simulink model "Turtle_RRT_Algorithm"  (R2023a)
settings: Solver=FixedStepDiscrete  StartTime=0.0  StopTime=Inf  FixedStep=0.01  RelTol=1e-3  EnableMultiTasking=on
model workspace (MAT data in the model file):
  SL_ROS_VariableLengthArrays_MaxSizes.CommonInfo.ArrayTruncateAction = 'EmitWarning'
  SL_ROS_VariableLengthArrays_MaxSizes.MsgTypeMap = containers.Map
  SL_ROS_VariableLengthArrays_MaxSizes.MsgTypeMap.serialization.keys = {'sensor_msgs/LaserScan'}
  SL_ROS_VariableLengthArrays_MaxSizes.MsgTypeMap.serialization.values{1}(1).PropertyName = 'Intensities'
  SL_ROS_VariableLengthArrays_MaxSizes.MsgTypeMap.serialization.values{1}(1).DataType = 'single'
  SL_ROS_VariableLengthArrays_MaxSizes.MsgTypeMap.serialization.values{1}(1).MaxLength = 360
  SL_ROS_VariableLengthArrays_MaxSizes.MsgTypeMap.serialization.values{1}(2).PropertyName = 'Ranges'
  SL_ROS_VariableLengthArrays_MaxSizes.MsgTypeMap.serialization.values{1}(2).DataType = 'single'
  SL_ROS_VariableLengthArrays_MaxSizes.MsgTypeMap.serialization.values{1}(2).MaxLength = 360
  SL_ROS_VariableLengthArrays_MaxSizes.MsgTypeMap.serialization.uniformity = 0
  SL_ROS_VariableLengthArrays_MaxSizes.MsgTypeMap.serialization.keyType = 'char'
  SL_ROS_VariableLengthArrays_MaxSizes.MsgTypeMap.serialization.valueType = 'any'
undefined symbols (not defined in the file or in its folder): Angular, gray, Linear
libraries: visiontextngfix x10, robotlib x6, simulink x4
settings Model: Creator=The MathWorks, Inc.  LastModifiedBy=cesf9
settings SolverCC: AlgebraicLoopSolver=TrustRegion
settings DataIOCC: LimitDataPoints=on  SaveFormat=Array  ReturnWorkspaceOutputs=off
settings OptimizationCC: LifeSpan=Inf  MaxStackSize=64
settings DebuggingCC: SolverPrmCheckMsg=warning  MultiTaskRateTransMsg=warning  UnconnectedInputMsg=warning  UnconnectedOutputMsg=warning  UnconnectedLineMsg=warning  SFUnexpectedBacktrackingDiag=warning  SFNoUnconditionalDefaultTransitionDiag=warning  SFExecutionAtInitializationDiag=none  ArithmeticOperatorsInVariantConditions=warning
settings HardwareCC: ProdBitPerPointer=32  ProdBitPerSizeT=32  ProdBitPerPtrDiffT=32  ProdLargestAtomicFloat=None  ProdIntDivRoundTo=Undefined  ProdEndianess=Unspecified  ProdWordSize=32  ProdHWDeviceType=Generic->Unspecified (assume 32-bit Generic)  UseEmbeddedCoderFeatures=off
settings ModelReferenceCC: EnableRefExpFcnMdlSchedulingChecks=on  PropagateSignalLabelsOutOfModel=off
settings SFSimCC: SimUseLocalCustomCode=off  SimTargetLang=C++
settings RTWCC: Description=Embedded Coder  SystemTargetFile=ert.tlc  HardwareBoard=Robot Operating System (ROS)  TLCOptions=-aInlineSetEventsForThisBaseRateFcn=TLC_FALSE -aSuppressMultiTaskScheduler=TLC_FALSE -aRateBasedStepFcn=0  TemplateMakefile=ert_default_tmf  RTWUseLocalCustomCode=off  Toolchain=Catkin  TargetLang=C++
settings CodeAppCC: StateflowObjectComments=on
settings ERTTargetCC: MultiwordLength=2048  ERTCustomFileBanners=off  SupportContinuousTime=on  SupportNonInlinedSFcns=on  RemoveResetFunc=off  SupportVariableSizeSignals=on  ModelStepFunctionPrototypeControlCompliant=off  ConvertIfToSwitch=off  SuppressUnreachableDefaultCases=off
settings ConfigComp: CovMetricSettings=dw  CovSaveCumulativeToWorkspaceVar=on  CovSaveSingleToWorkspaceVar=on  CovExternalEMLEnable=off  CovSFcnEnable=off

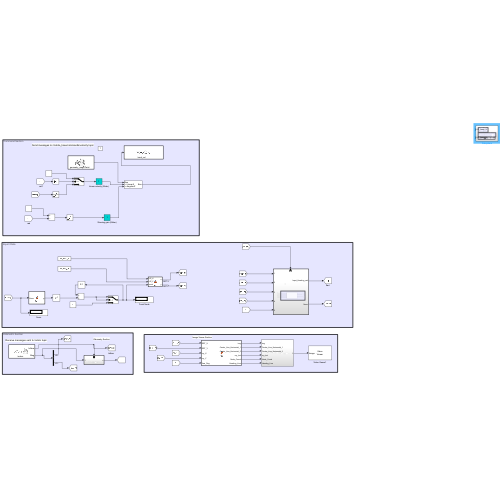
[thumbnail: Simulink's stored preview of the top-level diagram]
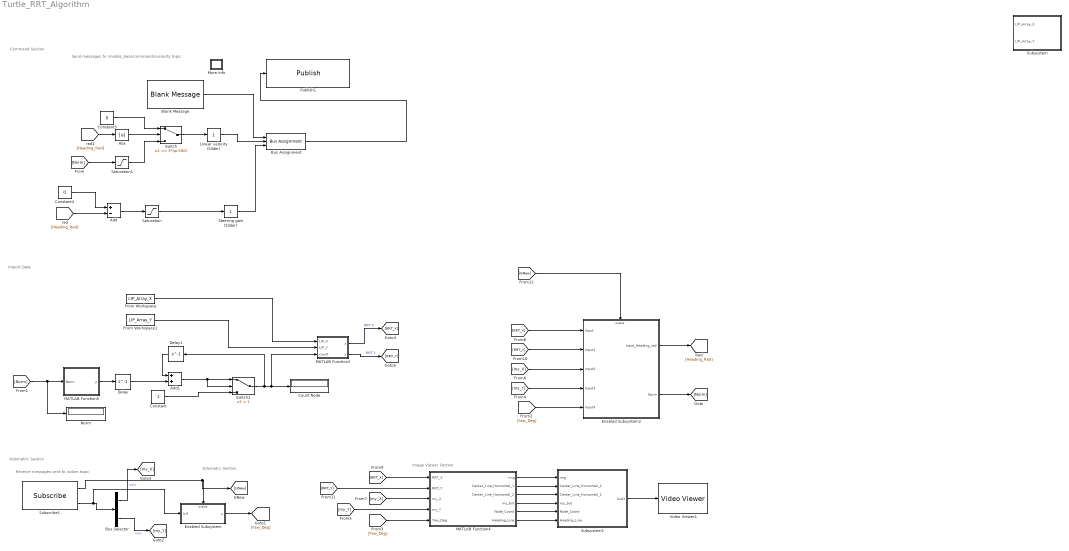
== system Turtle_RRT_Algorithm ==
  note: Image Viewer Section
  note: Import Data
  note: Odometry Section
  note: Odometric Section
  note: Command Section
  note: Receive messages sent to /odom topic
  note: Send messages to /mobile_base/commands/velocity topic
  Abs : Abs  SaturateOnIntegerOverflow=off
  Add : Sum  Inputs=+-
  Add1 : Sum
  Blank Message : robotlib/Blank Message  messageClass=Message  entityType=geometry_msgs/Twist  messageType=geometry_msgs/Twist  SampleTime=0.01  legacyBusStruct=off
  Bus Assignment : BusAssignment  DialogController=Simulink.DDGSource_BusAssignment  AssignedSignals=Linear.X,Angular.Z
  Bus Selector : BusSelector  DialogController=Simulink.DDGSource_BusSelector  OutputSignals=Pose.Pose.Position.X,Pose.Pose.Position.Y
  Constant : Constant
  Constant3 : Constant  Value=0
  Constant4 : Constant  Value=0
  Count Node : Display
  Delay : Delay  DelayLength=1
  Delay1 : Delay  DelayLength=1
  Enabled Subsystem : Subsystem  TreatAsAtomicUnit=on
  Enabled Subsystem2 : Subsystem  TreatAsAtomicUnit=on
  From Workspace : FromWorkspace  VariableName=LIP_Array_X  SampleTime=1
  From Workspace1 : FromWorkspace  VariableName=LIP_Array_Y  SampleTime=1
  Linear velocity (Slider) : simulink/Math Operations/Slider Gain  gain=1  low=0  high=2
  MATLAB Function2 : MATLAB Function  TreatAsAtomicUnit=on
  MATLAB Function4 : MATLAB Function  TreatAsAtomicUnit=on
  MATLAB Function5 : MATLAB Function  TreatAsAtomicUnit=on
  More Info : Subsystem
      settings: OpenFcn=showdemo(bdroot(gcb))
      mask Display: disp('?')
  Norm : Display
  Publish1 : robotlib/Publish  topicSource=Select from ROS network  topic=/cmd_vel  messageType=geometry_msgs/Twist  legacyBusStruct=off  messageQueueLength=105
  Saturation : Saturate  UpperLimit=0.3  LowerLimit=-0.3
  Saturation1 : Saturate  UpperLimit=0.3  LowerLimit=-0.3
  Steering gain (Slider) : simulink/Math Operations/Slider Gain  gain=1  low=-1  high=1
  Subscribe1 : robotlib/Subscribe  topicSource=Select from ROS network  topic=/odom  messageType=nav_msgs/Odometry  SampleTime=-1  legacyBusStruct=off  messageQueueLength=51
  Subsystem : Subsystem
  Subsystem1 : Subsystem
  Switch : Switch  Threshold=5*(pi/180)  SaturateOnIntegerOverflow=off  InputSameDT=off
  Switch1 : Switch  Criteria=u2 > Threshold  Threshold=1  SaturateOnIntegerOverflow=off  InputSameDT=off
  Video Viewer1 : VideoViewer  colormapValue=gray(256)  FigPos=[138 1038 776 784]
  wires:
  Subscribe1/2 -> Enabled Subsystem/1(In3), Bus Selector/1
  Subscribe1/1 -> [IsNew], Enabled Subsystem/Enable
  Steering gain (Slider)/1 -> Bus Assignment/3
  Bus Assignment/1 -> Publish1/1
  Blank Message/1 -> Bus Assignment/1
  Linear velocity (Slider)/1 -> Bus Assignment/2
  From Workspace/1 -> MATLAB Function2/1(LIP_X)
  From Workspace1/1 -> MATLAB Function2/2(LIP_Y)
  Switch/1 -> Linear velocity (Slider)/1
  MATLAB Function4/1(img) -> Subsystem1/1(img)
  MATLAB Function4/2(Center_Line_Horizontal_1) -> Subsystem1/2(Center_Line_Horizontal_1)
  MATLAB Function4/3(Center_Line_Horizontal_2) -> Subsystem1/3(Center_Line_Horizontal_2)
  MATLAB Function4/4(my_bot) -> Subsystem1/4(my_bot)
  MATLAB Function4/5(Node_Coord) -> Subsystem1/5(Node_Coord)
  Subsystem1/1(Out1) -> Video Viewer1/1
  MATLAB Function4/6(Heading_Line) -> Subsystem1/6(Heading_Line)
  Saturation/1 -> Steering gain (Slider)/1
  Constant4/1 -> Add/1
  Add/1 -> Saturation/1
  MATLAB Function5/1(p) -> Delay/1
  Delay/1 -> Add1/2
  Add1/1 -> Switch1/1, Switch1/2
  Constant/1 -> Switch1/3
  Switch1/1 -> MATLAB Function2/3(count), Count Node/1, Delay1/1
  Delay1/1 -> Add1/1
  Abs/1 -> Switch/2
  [Heading_Rad] -> Add/2
  [Norm] -> Saturation1/1
  [Norm] -> Norm/1, MATLAB Function5/1(Norm)
  Enabled Subsystem/1(u) -> [Yaw_Deg]
  [Yaw_Deg] -> MATLAB Function4/5(Yaw_Deg)
  Bus Selector/2 -> [my_Y]  "<Y>"
  [my_Y] -> MATLAB Function4/4(my_Y)
  Bus Selector/1 -> [my_X]  "<X>"
  [my_X] -> MATLAB Function4/3(my_X)
  MATLAB Function2/1(x) -> [RRT_X]  "RRT X"
  [RRT_X] -> MATLAB Function4/1(RRT_X)
  MATLAB Function2/2(y) -> [RRT_Y]  "RRT Y"
  [RRT_Y] -> MATLAB Function4/2(RRT_Y)
  Enabled Subsystem2/1(Input_Heading_rad) -> [Heading_Rad]
  Enabled Subsystem2/2(Norm) -> [Norm]
  [RRT_X] -> Enabled Subsystem2/1(Input)
  [RRT_Y] -> Enabled Subsystem2/2(Input1)
  [my_X] -> Enabled Subsystem2/3(Input2)
  [my_Y] -> Enabled Subsystem2/4(Input3)
  [Yaw_Deg] -> Enabled Subsystem2/5(Input4)
  [IsNew] -> Enabled Subsystem2/Enable
  [Heading_Rad] -> Abs/1
  Saturation1/1 -> Switch/3
  Constant3/1 -> Switch/1

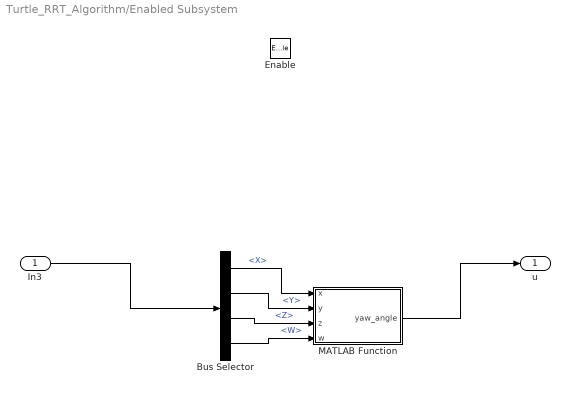
== system Turtle_RRT_Algorithm/Enabled Subsystem ==
  In3 : Inport
  Enable : EnablePort
  Bus Selector : BusSelector  OutputSignals=Pose.Pose.Orientation.X,Pose.Pose.Orientation.Y,Pose.Pose.Orientation.Z,Pose.Pose.Orientation.W
  MATLAB Function : MATLAB Function  TreatAsAtomicUnit=on
  u : Outport
  wires:
  In3/1 -> Bus Selector/1
  Bus Selector/1 -> MATLAB Function/1(x)  "<X>"
  Bus Selector/2 -> MATLAB Function/2(y)  "<Y>"
  Bus Selector/3 -> MATLAB Function/3(z)  "<Z>"
  Bus Selector/4 -> MATLAB Function/4(w)  "<W>"
  MATLAB Function/1(yaw_angle) -> u/1

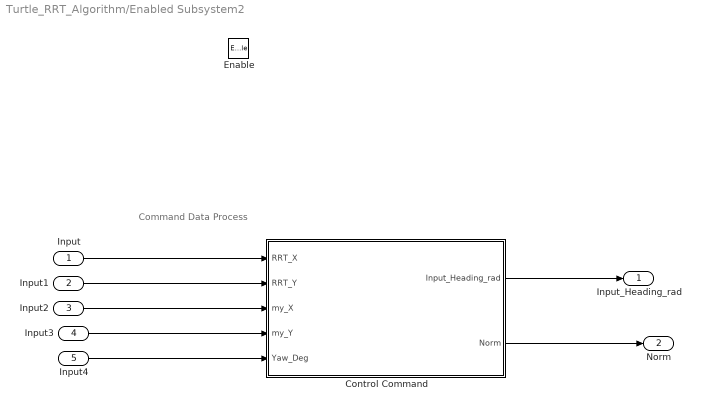
== system Turtle_RRT_Algorithm/Enabled Subsystem2 ==
  note: Command Data Process
  Input : Inport
  Input1 : Inport  Port=2
  Input2 : Inport  Port=3
  Input3 : Inport  Port=4
  Input4 : Inport  Port=5
  Enable : EnablePort
  Control Command : MATLAB Function  TreatAsAtomicUnit=on
  Input_Heading_rad : Outport
  Norm : Outport  Port=2
  wires:
  Control Command/1(Input_Heading_rad) -> Input_Heading_rad/1
  Input4/1 -> Control Command/5(Yaw_Deg)
  Input2/1 -> Control Command/3(my_X)
  Control Command/2(Norm) -> Norm/1
  Input/1 -> Control Command/1(RRT_X)
  Input3/1 -> Control Command/4(my_Y)
  Input1/1 -> Control Command/2(RRT_Y)

== system Turtle_RRT_Algorithm/More Info ==

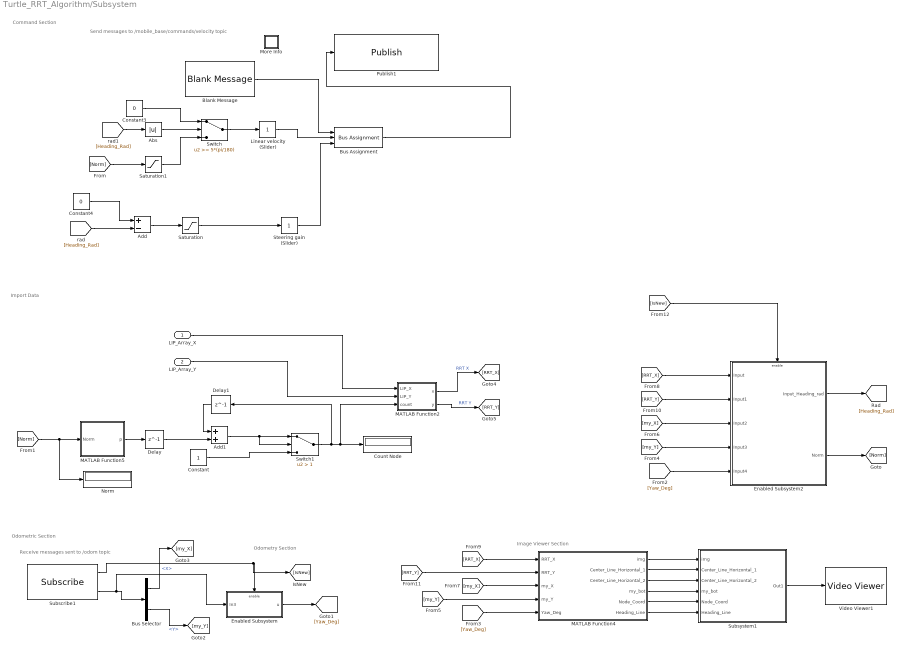
== system Turtle_RRT_Algorithm/Subsystem ==
  note: Command Section
  note: Odometry Section
  note: Image Viewer Section
  note: Import Data
  note: Odometric Section
  note: Receive messages sent to /odom topic
  note: Send messages to /mobile_base/commands/velocity topic
  LIP_Array_X : Inport
  LIP_Array_Y : Inport  Port=2
  Abs : Abs  SaturateOnIntegerOverflow=off
  Add : Sum  Inputs=+-
  Add1 : Sum
  Blank Message : robotlib/Blank Message  messageClass=Message  entityType=geometry_msgs/Twist  messageType=geometry_msgs/Twist  SampleTime=0.01  legacyBusStruct=off
  Bus Assignment : BusAssignment  DialogController=Simulink.DDGSource_BusAssignment  AssignedSignals=Linear.X,Angular.Z
  Bus Selector : BusSelector  DialogController=Simulink.DDGSource_BusSelector  OutputSignals=Pose.Pose.Position.X,Pose.Pose.Position.Y
  Constant : Constant
  Constant3 : Constant  Value=0
  Constant4 : Constant  Value=0
  Count Node : Display
  Delay : Delay  DelayLength=1
  Delay1 : Delay  DelayLength=1
  Enabled Subsystem : Subsystem  TreatAsAtomicUnit=on
  Enabled Subsystem2 : Subsystem  TreatAsAtomicUnit=on
  Linear velocity (Slider) : simulink/Math Operations/Slider Gain  gain=1  low=0  high=2
  MATLAB Function2 : MATLAB Function  TreatAsAtomicUnit=on
  MATLAB Function4 : MATLAB Function  TreatAsAtomicUnit=on
  MATLAB Function5 : MATLAB Function  TreatAsAtomicUnit=on
  More Info : Subsystem
      settings: OpenFcn=showdemo(bdroot(gcb))
      mask Display: disp('?')
  Norm : Display
  Publish1 : robotlib/Publish  topicSource=Select from ROS network  topic=/cmd_vel  messageType=geometry_msgs/Twist  legacyBusStruct=off  messageQueueLength=105
  Saturation : Saturate  UpperLimit=0.3  LowerLimit=-0.3
  Saturation1 : Saturate  UpperLimit=0.3  LowerLimit=-0.3
  Steering gain (Slider) : simulink/Math Operations/Slider Gain  gain=1  low=-1  high=1
  Subscribe1 : robotlib/Subscribe  topicSource=Select from ROS network  topic=/odom  messageType=nav_msgs/Odometry  SampleTime=-1  legacyBusStruct=off  messageQueueLength=51
  Subsystem1 : Subsystem
  Switch : Switch  Threshold=5*(pi/180)  SaturateOnIntegerOverflow=off  InputSameDT=off
  Switch1 : Switch  Criteria=u2 > Threshold  Threshold=1  SaturateOnIntegerOverflow=off  InputSameDT=off
  Video Viewer1 : VideoViewer  colormapValue=gray(256)  FigPos=[138 1038 776 784]
  wires:
  Saturation/1 -> Steering gain (Slider)/1
  Subsystem1/1(Out1) -> Video Viewer1/1
  [Norm] -> Saturation1/1
  [Heading_Rad] -> Add/2
  Enabled Subsystem/1(u) -> [Yaw_Deg]
  Delay1/1 -> Add1/1
  MATLAB Function4/1(img) -> Subsystem1/1(img)
  Bus Selector/2 -> [my_Y]  "<Y>"
  [Yaw_Deg] -> MATLAB Function4/5(Yaw_Deg)
  Add/1 -> Saturation/1
  Subscribe1/2 -> Enabled Subsystem/1(In3), Bus Selector/1
  Steering gain (Slider)/1 -> Bus Assignment/3
  Switch/1 -> Linear velocity (Slider)/1
  Bus Assignment/1 -> Publish1/1
  MATLAB Function4/5(Node_Coord) -> Subsystem1/5(Node_Coord)
  [my_X] -> Enabled Subsystem2/3(Input2)
  Blank Message/1 -> Bus Assignment/1
  MATLAB Function4/4(my_bot) -> Subsystem1/4(my_bot)
  LIP_Array_X/1 -> MATLAB Function2/1(LIP_X)
  MATLAB Function4/3(Center_Line_Horizontal_2) -> Subsystem1/3(Center_Line_Horizontal_2)
  Bus Selector/1 -> [my_X]  "<X>"
  MATLAB Function5/1(p) -> Delay/1
  Add1/1 -> Switch1/1, Switch1/2
  [my_X] -> MATLAB Function4/3(my_X)
  [RRT_X] -> MATLAB Function4/1(RRT_X)
  Enabled Subsystem2/2(Norm) -> [Norm]
  [my_Y] -> MATLAB Function4/4(my_Y)
  [Norm] -> Norm/1, MATLAB Function5/1(Norm)
  MATLAB Function2/2(y) -> [RRT_Y]  "RRT Y"
  Enabled Subsystem2/1(Input_Heading_rad) -> [Heading_Rad]
  Delay/1 -> Add1/2
  [IsNew] -> Enabled Subsystem2/Enable
  Subscribe1/1 -> [IsNew], Enabled Subsystem/Enable
  Saturation1/1 -> Switch/3
  Constant/1 -> Switch1/3
  MATLAB Function4/6(Heading_Line) -> Subsystem1/6(Heading_Line)
  [Yaw_Deg] -> Enabled Subsystem2/5(Input4)
  LIP_Array_Y/1 -> MATLAB Function2/2(LIP_Y)
  MATLAB Function2/1(x) -> [RRT_X]  "RRT X"
  Switch1/1 -> MATLAB Function2/3(count), Count Node/1, Delay1/1
  Linear velocity (Slider)/1 -> Bus Assignment/2
  [RRT_X] -> Enabled Subsystem2/1(Input)
  [Heading_Rad] -> Abs/1
  Constant4/1 -> Add/1
  Abs/1 -> Switch/2
  [my_Y] -> Enabled Subsystem2/4(Input3)
  Constant3/1 -> Switch/1
  [RRT_Y] -> Enabled Subsystem2/2(Input1)
  MATLAB Function4/2(Center_Line_Horizontal_1) -> Subsystem1/2(Center_Line_Horizontal_1)
  [RRT_Y] -> MATLAB Function4/2(RRT_Y)

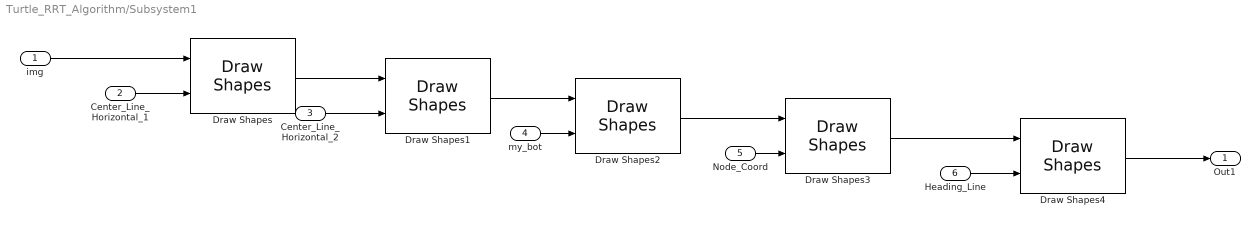
== system Turtle_RRT_Algorithm/Subsystem1 ==
  img : Inport
  Center_Line_Horizontal_1 : Inport  Port=2
  Center_Line_Horizontal_2 : Inport  Port=3
  my_bot : Inport  Port=4
  Node_Coord : Inport  Port=5
  Heading_Line : Inport  Port=6
  Draw Shapes : visiontextngfix/Draw Shapes  shape=Lines  fill=off  lineWidth=1  fillClrSource=Specify via dialog  display=Black  intensity=200  color=[255 0 0]  opacity=0.6  viewport=Entire image  antialiasing=off  inType=Obsolete  imagePorts=One multidimensional signal  roundingMode=Floor  overflowMode=off  memoryMode=Specify word length  memoryWordLength=16  prodOutputMode=Binary point scaling  prodOutputWordLength=32  prodOutputFracLength=14  memoryFracLength=15
  Draw Shapes1 : visiontextngfix/Draw Shapes  shape=Lines  fill=off  lineWidth=1  fillClrSource=Specify via dialog  display=Black  intensity=200  color=[200 255 100]  opacity=0.6  viewport=Entire image  antialiasing=off  inType=Obsolete  imagePorts=One multidimensional signal  roundingMode=Floor  overflowMode=off  memoryMode=Specify word length  memoryWordLength=16  prodOutputMode=Binary point scaling  prodOutputWordLength=32  prodOutputFracLength=14  memoryFracLength=15
  Draw Shapes2 : visiontextngfix/Draw Shapes  shape=Circles  fill=off  lineWidth=3  fillClrSource=Specify via dialog  display=Black  intensity=200  color=[200 255 100]  opacity=0.6  viewport=Entire image  antialiasing=off  inType=Obsolete  imagePorts=One multidimensional signal  roundingMode=Floor  overflowMode=off  memoryMode=Specify word length  memoryWordLength=16  prodOutputMode=Binary point scaling  prodOutputWordLength=32  prodOutputFracLength=14  memoryFracLength=15
  Draw Shapes3 : visiontextngfix/Draw Shapes  shape=Circles  fill=on  lineWidth=1  fillClrSource=Specify via dialog  display=Black  intensity=200  color=[200 255 100]  opacity=0.6  viewport=Entire image  antialiasing=off  inType=Obsolete  imagePorts=One multidimensional signal  roundingMode=Floor  overflowMode=off  memoryMode=Specify word length  memoryWordLength=16  prodOutputMode=Binary point scaling  prodOutputWordLength=32  prodOutputFracLength=14  memoryFracLength=15
  Draw Shapes4 : visiontextngfix/Draw Shapes  shape=Lines  fill=off  lineWidth=1  fillClrSource=Specify via dialog  display=Black  intensity=200  color=[200 255 100]  opacity=0.6  viewport=Entire image  antialiasing=off  inType=Obsolete  imagePorts=One multidimensional signal  roundingMode=Floor  overflowMode=off  memoryMode=Specify word length  memoryWordLength=16  prodOutputMode=Binary point scaling  prodOutputWordLength=32  prodOutputFracLength=14  memoryFracLength=15
  Out1 : Outport
  wires:
  Draw Shapes1/1 -> Draw Shapes2/1
  Node_Coord/1 -> Draw Shapes3/2
  Draw Shapes/1 -> Draw Shapes1/1
  Draw Shapes2/1 -> Draw Shapes3/1
  Draw Shapes3/1 -> Draw Shapes4/1
  Center_Line_Horizontal_2/1 -> Draw Shapes1/2
  Center_Line_Horizontal_1/1 -> Draw Shapes/2
  my_bot/1 -> Draw Shapes2/2
  img/1 -> Draw Shapes/1
  Heading_Line/1 -> Draw Shapes4/2
  Draw Shapes4/1 -> Out1/1

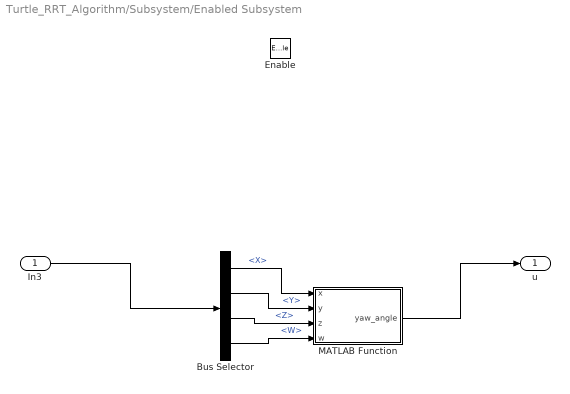
== system Turtle_RRT_Algorithm/Subsystem/Enabled Subsystem ==
  In3 : Inport
  Enable : EnablePort
  Bus Selector : BusSelector  OutputSignals=Pose.Pose.Orientation.X,Pose.Pose.Orientation.Y,Pose.Pose.Orientation.Z,Pose.Pose.Orientation.W
  MATLAB Function : MATLAB Function  TreatAsAtomicUnit=on
  u : Outport
  wires:
  In3/1 -> Bus Selector/1
  Bus Selector/1 -> MATLAB Function/1(x)  "<X>"
  Bus Selector/2 -> MATLAB Function/2(y)  "<Y>"
  Bus Selector/3 -> MATLAB Function/3(z)  "<Z>"
  Bus Selector/4 -> MATLAB Function/4(w)  "<W>"
  MATLAB Function/1(yaw_angle) -> u/1

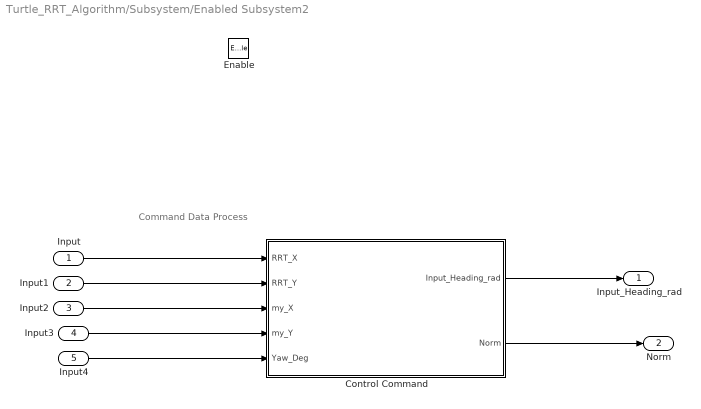
== system Turtle_RRT_Algorithm/Subsystem/Enabled Subsystem2 ==
  note: Command Data Process
  Input : Inport
  Input1 : Inport  Port=2
  Input2 : Inport  Port=3
  Input3 : Inport  Port=4
  Input4 : Inport  Port=5
  Enable : EnablePort
  Control Command : MATLAB Function  TreatAsAtomicUnit=on
  Input_Heading_rad : Outport
  Norm : Outport  Port=2
  wires:
  Control Command/1(Input_Heading_rad) -> Input_Heading_rad/1
  Input4/1 -> Control Command/5(Yaw_Deg)
  Input2/1 -> Control Command/3(my_X)
  Control Command/2(Norm) -> Norm/1
  Input/1 -> Control Command/1(RRT_X)
  Input3/1 -> Control Command/4(my_Y)
  Input1/1 -> Control Command/2(RRT_Y)

== system Turtle_RRT_Algorithm/Subsystem/More Info ==

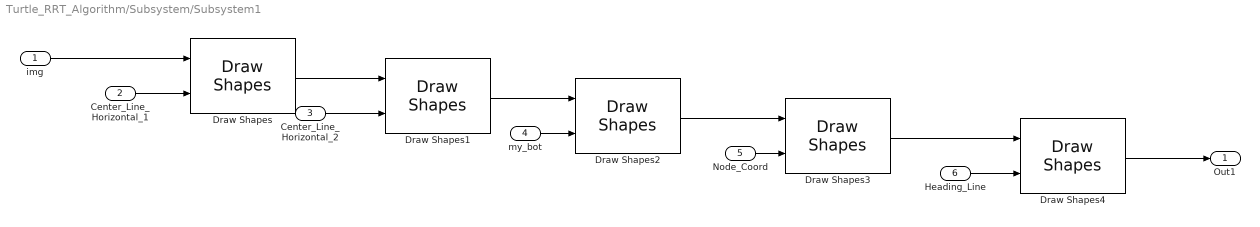
== system Turtle_RRT_Algorithm/Subsystem/Subsystem1 ==
  img : Inport
  Center_Line_Horizontal_1 : Inport  Port=2
  Center_Line_Horizontal_2 : Inport  Port=3
  my_bot : Inport  Port=4
  Node_Coord : Inport  Port=5
  Heading_Line : Inport  Port=6
  Draw Shapes : visiontextngfix/Draw Shapes  shape=Lines  fill=off  lineWidth=1  fillClrSource=Specify via dialog  display=Black  intensity=200  color=[255 0 0]  opacity=0.6  viewport=Entire image  antialiasing=off  inType=Obsolete  imagePorts=One multidimensional signal  roundingMode=Floor  overflowMode=off  memoryMode=Specify word length  memoryWordLength=16  prodOutputMode=Binary point scaling  prodOutputWordLength=32  prodOutputFracLength=14  memoryFracLength=15
  Draw Shapes1 : visiontextngfix/Draw Shapes  shape=Lines  fill=off  lineWidth=1  fillClrSource=Specify via dialog  display=Black  intensity=200  color=[200 255 100]  opacity=0.6  viewport=Entire image  antialiasing=off  inType=Obsolete  imagePorts=One multidimensional signal  roundingMode=Floor  overflowMode=off  memoryMode=Specify word length  memoryWordLength=16  prodOutputMode=Binary point scaling  prodOutputWordLength=32  prodOutputFracLength=14  memoryFracLength=15
  Draw Shapes2 : visiontextngfix/Draw Shapes  shape=Circles  fill=off  lineWidth=3  fillClrSource=Specify via dialog  display=Black  intensity=200  color=[200 255 100]  opacity=0.6  viewport=Entire image  antialiasing=off  inType=Obsolete  imagePorts=One multidimensional signal  roundingMode=Floor  overflowMode=off  memoryMode=Specify word length  memoryWordLength=16  prodOutputMode=Binary point scaling  prodOutputWordLength=32  prodOutputFracLength=14  memoryFracLength=15
  Draw Shapes3 : visiontextngfix/Draw Shapes  shape=Circles  fill=on  lineWidth=1  fillClrSource=Specify via dialog  display=Black  intensity=200  color=[200 255 100]  opacity=0.6  viewport=Entire image  antialiasing=off  inType=Obsolete  imagePorts=One multidimensional signal  roundingMode=Floor  overflowMode=off  memoryMode=Specify word length  memoryWordLength=16  prodOutputMode=Binary point scaling  prodOutputWordLength=32  prodOutputFracLength=14  memoryFracLength=15
  Draw Shapes4 : visiontextngfix/Draw Shapes  shape=Lines  fill=off  lineWidth=1  fillClrSource=Specify via dialog  display=Black  intensity=200  color=[200 255 100]  opacity=0.6  viewport=Entire image  antialiasing=off  inType=Obsolete  imagePorts=One multidimensional signal  roundingMode=Floor  overflowMode=off  memoryMode=Specify word length  memoryWordLength=16  prodOutputMode=Binary point scaling  prodOutputWordLength=32  prodOutputFracLength=14  memoryFracLength=15
  Out1 : Outport
  wires:
  Draw Shapes1/1 -> Draw Shapes2/1
  Node_Coord/1 -> Draw Shapes3/2
  Draw Shapes/1 -> Draw Shapes1/1
  Draw Shapes2/1 -> Draw Shapes3/1
  Draw Shapes3/1 -> Draw Shapes4/1
  Center_Line_Horizontal_2/1 -> Draw Shapes1/2
  Center_Line_Horizontal_1/1 -> Draw Shapes/2
  my_bot/1 -> Draw Shapes2/2
  img/1 -> Draw Shapes/1
  Heading_Line/1 -> Draw Shapes4/2
  Draw Shapes4/1 -> Out1/1

== matlab function Turtle_RRT_Algorithm/MATLAB Function5 ==
  data: p output; Norm input
function p = fcn(Norm)
p = 0;

if Norm < 0.5
    p = 1;
end

== matlab function Turtle_RRT_Algorithm/Enabled Subsystem2/Control Command ==
  data: RRT_X input; RRT_Y input; my_X input; my_Y input; Yaw_Deg input; Input_Heading_rad output; Norm output
function [Input_Heading_rad,Norm]  = fcn(RRT_X, RRT_Y, my_X, my_Y, Yaw_Deg)

Vector = zeros(1,2);

Vector(1,1) = RRT_X - my_X;
Vector(1,2) = RRT_Y - my_Y;

Norm = norm(Vector);

Com_Vector = complex(Vector(1,1), Vector(1,2));

Heading_Rad = angle(Com_Vector);

Heading_Deg = rad2deg(Heading_Rad);

Ref_Heading = Yaw_Deg - Heading_Deg;

Input_Heading = 0;

if Ref_Heading > 180
    Input_Heading = Ref_Heading - 360;
elseif Ref_Heading < -180
    Input_Heading = 360 - Ref_Heading;
else
    Input_Heading = Ref_Heading;
end

Input_Heading_rad = (2*pi/360)*Input_Heading;


% coder.extrinsic('polarplot');
% 
% X = [my_X RRT_X];
% Y = [my_Y RRT_Y];
% 
% color = [1 7];
% 
% figure(2)
% scatter(X,Y,25,color,'filled');
% axis([-10 10 -10 10])

== matlab function Turtle_RRT_Algorithm/Subsystem/Enabled Subsystem/MATLAB Function ==
  data: x input; yaw_angle output; y input; z input; w input
function yaw_angle  = fcn(x, y, z, w)

quat = [w x y z];
eul_angle = quat2eul(quat);
yaw_angle = rad2deg(eul_angle(1));

== matlab function Turtle_RRT_Algorithm/Subsystem/Enabled Subsystem2/Control Command ==
  data: RRT_X input; RRT_Y input; my_X input; my_Y input; Yaw_Deg input; Input_Heading_rad output; Norm output
function [Input_Heading_rad,Norm]  = fcn(RRT_X, RRT_Y, my_X, my_Y, Yaw_Deg)

Vector = zeros(1,2);

Vector(1,1) = RRT_X - my_X;
Vector(1,2) = RRT_Y - my_Y;

Norm = norm(Vector);

Com_Vector = complex(Vector(1,1), Vector(1,2));

Heading_Rad = angle(Com_Vector);

Heading_Deg = rad2deg(Heading_Rad);

Ref_Heading = Yaw_Deg - Heading_Deg;

Input_Heading = 0;

if Ref_Heading > 180
    Input_Heading = Ref_Heading - 360;
elseif Ref_Heading < -180
    Input_Heading = 360 - Ref_Heading;
else
    Input_Heading = Ref_Heading;
end

Input_Heading_rad = (2*pi/360)*Input_Heading;


% coder.extrinsic('polarplot');
% 
% X = [my_X RRT_X];
% Y = [my_Y RRT_Y];
% 
% color = [1 7];
% 
% figure(2)
% scatter(X,Y,25,color,'filled');
% axis([-10 10 -10 10])

== matlab function Turtle_RRT_Algorithm/Subsystem/MATLAB Function2 ==
  data: x output; LIP_X input; LIP_Y input; y output; count input
function [x,y] = fcn(LIP_X, LIP_Y, count)

x = LIP_X(count,1);
y = LIP_Y(count,1);

== matlab function Turtle_RRT_Algorithm/Subsystem/MATLAB Function4 ==
  data: RRT_X input; img output; RRT_Y input; my_X input; my_Y input; Center_Line_Horizontal_1 output; Center_Line_Horizontal_2 output; my_bot output; Node_Coord output; Yaw_Deg input; Heading_Line output
function [img,Center_Line_Horizontal_1,Center_Line_Horizontal_2,my_bot,Node_Coord,Heading_Line] = fcn(RRT_X, RRT_Y, my_X, my_Y, Yaw_Deg)

img = ones(2048);

center = 2048/2;

Center_Line_Horizontal_1 = [center 1 center 2048];
Center_Line_Horizontal_2 = [1 center 2048 center];

my_col = center - my_Y;
my_row = center + my_X;

Node_col = center - RRT_Y;
Node_row = center + RRT_X;

my_bot = [my_row ,my_col,3; my_row,my_col,1];
Node_Coord = [Node_row, Node_col, 5; Node_row, Node_col, 2];

Yaw_Rad = deg2rad(Yaw_Deg);

Heading_Angle_X = my_X + 10*cos(Yaw_Rad);
Heading_Angle_Y = my_Y + 10*sin(Yaw_Rad);

Heading_col = center - Heading_Angle_Y;
Heading_row = center + Heading_Angle_X;

Heading_Line = [my_row my_col Heading_row Heading_col];

== matlab function Turtle_RRT_Algorithm/Subsystem/MATLAB Function5 ==
  data: p output; Norm input
function p = fcn(Norm)
p = 0;

if Norm < 0.5
    p = 1;
end

== matlab function Turtle_RRT_Algorithm/MATLAB Function2 ==
  data: x output; LIP_X input; LIP_Y input; y output; count input
function [x,y] = fcn(LIP_X, LIP_Y, count)

x = LIP_X(count,1);
y = LIP_Y(count,1);

== matlab function Turtle_RRT_Algorithm/Enabled Subsystem/MATLAB Function ==
  data: x input; yaw_angle output; y input; z input; w input
function yaw_angle  = fcn(x, y, z, w)

quat = [w x y z];
eul_angle = quat2eul(quat);
yaw_angle = rad2deg(eul_angle(1));

== matlab function Turtle_RRT_Algorithm/MATLAB Function4 ==
  data: RRT_X input; img output; RRT_Y input; my_X input; my_Y input; Center_Line_Horizontal_1 output; Center_Line_Horizontal_2 output; my_bot output; Node_Coord output; Yaw_Deg input; Heading_Line output
function [img,Center_Line_Horizontal_1,Center_Line_Horizontal_2,my_bot,Node_Coord,Heading_Line] = fcn(RRT_X, RRT_Y, my_X, my_Y, Yaw_Deg)

img = ones(2048);

center = 2048/2;

Center_Line_Horizontal_1 = [center 1 center 2048];
Center_Line_Horizontal_2 = [1 center 2048 center];

my_col = center - my_Y;
my_row = center + my_X;

Node_col = center - RRT_Y;
Node_row = center + RRT_X;

my_bot = [my_row ,my_col,3; my_row,my_col,1];
Node_Coord = [Node_row, Node_col, 5; Node_row, Node_col, 2];

Yaw_Rad = deg2rad(Yaw_Deg);

Heading_Angle_X = my_X + 10*cos(Yaw_Rad);
Heading_Angle_Y = my_Y + 10*sin(Yaw_Rad);

Heading_col = center - Heading_Angle_Y;
Heading_row = center + Heading_Angle_X;

Heading_Line = [my_row my_col Heading_row Heading_col];
